simulink model "GliderSim"  (R2017a)
settings: Solver=ode4  StartTime=0.0  StopTime=10.0  FixedStep=0.01  RelTol=1e-3
libraries: simulink x1
settings Model: Creator=Caleb  LastModifiedBy=Caleb
settings DebuggingCC: AlgebraicLoopMsg=none

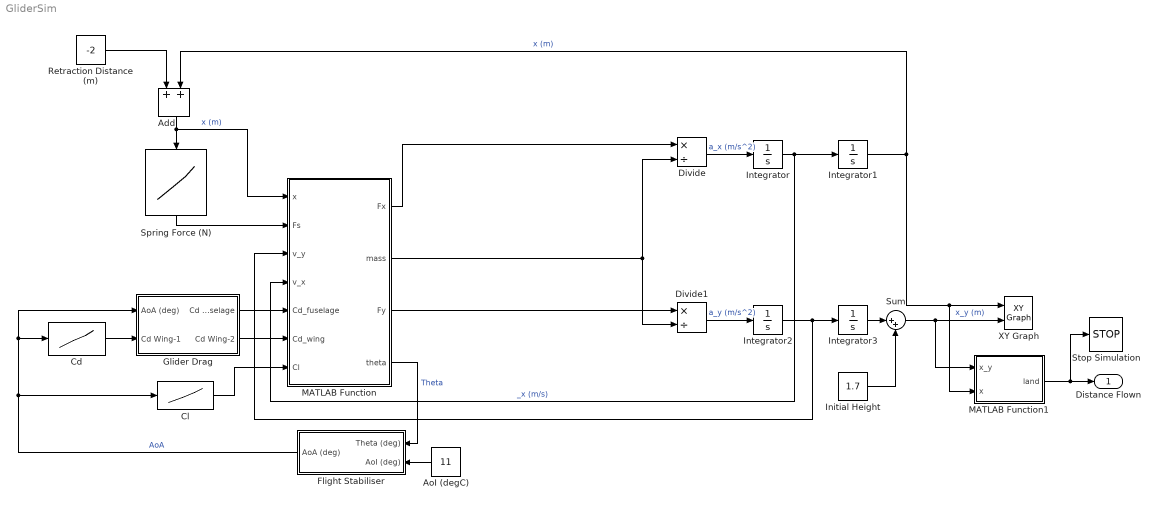
== system GliderSim ==
  Add : Sum
  AoI (degC) : Constant  Value=11
  Cd : Lookup_n-D  NumberOfTableDimensions=1  BreakpointsForDimension1="[-7.25           -7        -6.75         -6.5        -6.25           -6        -5.75         -5.5           -5        -4.75         -4.5        -4.25           -4        -3.75         -3.5        -3.25           -3        -2.75         -2.5        -2.25           -2        -1.75         -1.5        -1.25           -1        -0.75         -0.5        -0.25            0         0.25          0.5         0.75            1         1.25          1.5         1.75            2         2.25          2.5         2.75            3         3.25          3.5         3.75            4         4.25          4.5         4.75            5         5.25          5.5         5.75            6         6.25          6.5         6.75            7         7.25          7.5         7.75            8         8.25          8.5         8.75            9         9.25          9.5         9.75           10        10.25         10.5        10.75           11        11.25         11.5        11.75           12]"  Table="[0.09777      0.0974     0.09689     0.09609     0.09351     0.08904     0.08679     0.08458     0.07885     0.07578      0.0702      0.0665     0.06176     0.05768     0.05386     0.04963     0.04581     0.03137     0.02739     0.02531     0.02361     0.02247     0.02137     0.02112     0.02128     0.02105     0.02044      0.0201     0.01838     0.01859     0.01848     0.01875     0.01858     0.01891     0.01914     0.01911     0.01941     0.01899     0.01894     0.01863     0.01831     0.01814     0.01808     0.01797     0.01811     0.01819     0.01799     0.01697     0.01665     0.01637     0.01647     0.01697     0.01902     0.02138     0.02345     0.02462     0.02592     0.02747     0.02917     0.03059     0.03229      0.0344     0.03757     0.04309     0.04367     0.04789      0.0548     0.05508     0.05989     0.06817      0.0736     0.06647     0.07095      0.0758      0.0812     0.08707     0.09323]"  InternalRulePriority=Speed  RndMeth=Simplest  InputSameDT=on
  Cl : Lookup_n-D  NumberOfTableDimensions=1  BreakpointsForDimension1="[-7.25           -7        -6.75         -6.5        -6.25           -6        -5.75         -5.5           -5        -4.75         -4.5        -4.25           -4        -3.75         -3.5        -3.25           -3        -2.75         -2.5        -2.25           -2        -1.75         -1.5        -1.25           -1        -0.75         -0.5        -0.25            0         0.25          0.5         0.75            1         1.25          1.5         1.75            2         2.25          2.5         2.75            3         3.25          3.5         3.75            4         4.25          4.5         4.75            5         5.25          5.5         5.75            6         6.25          6.5         6.75            7         7.25          7.5         7.75            8         8.25          8.5         8.75            9         9.25          9.5         9.75           10        10.25         10.5        10.75           11        11.25         11.5        11.75           12]"  Table="[-0.3365     -0.3541     -0.3685     -0.3775     -0.3798     -0.3786     -0.3789     -0.3791     -0.3645     -0.3584     -0.3039     -0.2799      -0.238     -0.1968     -0.1591     -0.1118     -0.0705      0.0097      0.0582      0.0957      0.1363      0.1724       0.213       0.247      0.2882      0.3178      0.3638       0.393      0.4499      0.4792      0.5222      0.5478      0.5899      0.6131      0.6407      0.6755         0.7      0.7402      0.7667      0.7963      0.8258       0.854      0.8828      0.9128      0.9373      0.9628      0.9903      1.0184      1.0395      1.0579      1.0721      1.0813      1.0773      1.0773      1.0819      1.0965      1.1091      1.1174      1.1213      1.1304      1.1416      1.1651      1.2133      1.2732      1.2909       1.315       1.345        1.34      1.3474       1.347       1.319      1.2176      1.1873      1.1566      1.1247      1.0927      1.0614]"  InternalRulePriority=Speed  RndMeth=Simplest  InputSameDT=on
  Divide : Product  Inputs=*/
  Divide1 : Product  Inputs=*/
  Flight Stabiliser : Subsystem
  Glider Drag : Subsystem
  Initial Height : Constant  Value=1.7
  Integrator{,1..3} (4 alike) : Integrator
  MATLAB Function : MATLAB Function  TreatAsAtomicUnit=on
  MATLAB Function1 : MATLAB Function  TreatAsAtomicUnit=on
  Retraction Distance (m) : Constant  Value=-2
  Spring Force (N) : Lookup_n-D  NumberOfTableDimensions=1  BreakpointsForDimension1=[-2.16;-1.86;-1.62;-1.32;-1.00;-0.78;-0.42;-0.20;0;1]  Table=[75;62;56;48;40;33;23;13;0;0]  InternalRulePriority=Speed  RndMeth=Simplest  InputSameDT=on
  Stop Simulation : Stop
  Sum : Sum  Inputs=|++
  XY Graph : simulink/Sinks/XY Graph  xmin=0  xmax=70  ymin=0  ymax=5  st=-1
  Distance Flown : Outport
  wires:
  Add/1 -> MATLAB Function/1(x), Spring Force (N)/1  "x (m)"
  Divide/1 -> Integrator/1  "a_x (m/s^2)"
  Integrator/1 -> Integrator1/1, MATLAB Function/4(v_x)  "_x (m/s)"
  Integrator1/1 -> MATLAB Function1/2(x), XY Graph/1, Add/2  "x (m)"
  Retraction Distance (m)/1 -> Add/1
  Spring Force (N)/1 -> MATLAB Function/2(Fs)
  MATLAB Function/1(Fx) -> Divide/1
  MATLAB Function/2(mass) -> Divide/2, Divide1/2
  MATLAB Function/3(Fy) -> Divide1/1
  Divide1/1 -> Integrator2/1  "a_y (m/s^2)"
  Integrator2/1 -> Integrator3/1, MATLAB Function/3(v_y)
  Integrator3/1 -> Sum/1
  Initial Height/1 -> Sum/2
  Sum/1 -> XY Graph/2, MATLAB Function1/1(x_y)  "x_y (m)"
  MATLAB Function1/1(land) -> Stop Simulation/1, Distance Flown/1
  Flight Stabiliser/1(AoA (deg)) -> Glider Drag/1(AoA (deg)), Cd/1, Cl/1  "AoA"
  MATLAB Function/4(theta) -> Flight Stabiliser/1(Theta (deg))  "Theta"
  Cl/1 -> MATLAB Function/7(Cl)
  AoI (degC)/1 -> Flight Stabiliser/2(AoI (deg))
  Cd/1 -> Glider Drag/2(Cd Wing-1)
  Glider Drag/2(Cd Wing-2) -> MATLAB Function/6(Cd_wing)
  Glider Drag/1(Cd Fuselage) -> MATLAB Function/5(Cd_fuselage)

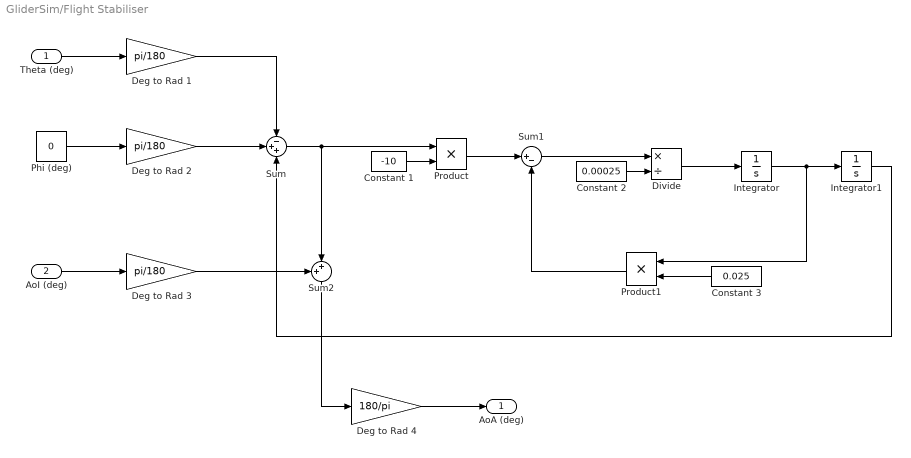
== system GliderSim/Flight Stabiliser ==
  Theta (deg) : Inport
  AoI (deg) : Inport  Port=2
  Constant 1 : Constant  Value=-10
  Constant 2 : Constant  Value=0.00025
  Constant 3 : Constant  Value=0.025
  Deg to Rad 1 : Gain  Gain=pi/180
  Deg to Rad 2 : Gain  Gain=pi/180
  Deg to Rad 3 : Gain  Gain=pi/180
  Deg to Rad 4 : Gain  Gain=180/pi
  Divide : Product  Inputs=*/
  Integrator : Integrator
  Integrator1 : Integrator
  Phi (deg) : Constant  Value=0
  Product : Product
  Product1 : Product
  Sum : Sum  Inputs=-++
  Sum1 : Sum  Inputs=|+-
  Sum2 : Sum  Inputs=++|
  AoA (deg) : Outport
  wires:
  Sum/1 -> Sum2/2, Product/1
  Divide/1 -> Integrator/1
  Integrator/1 -> Product1/1, Integrator1/1
  Sum1/1 -> Divide/1
  Deg to Rad 2/1 -> Sum/2
  Constant 1/1 -> Product/2
  Product/1 -> Sum1/1
  Constant 2/1 -> Divide/2
  Phi (deg)/1 -> Deg to Rad 2/1
  Sum2/1 -> Deg to Rad 4/1
  Deg to Rad 3/1 -> Sum2/1
  Theta (deg)/1 -> Deg to Rad 1/1
  AoI (deg)/1 -> Deg to Rad 3/1
  Product1/1 -> Sum1/2
  Integrator1/1 -> Sum/3
  Constant 3/1 -> Product1/2
  Deg to Rad 1/1 -> Sum/1
  Deg to Rad 4/1 -> AoA (deg)/1

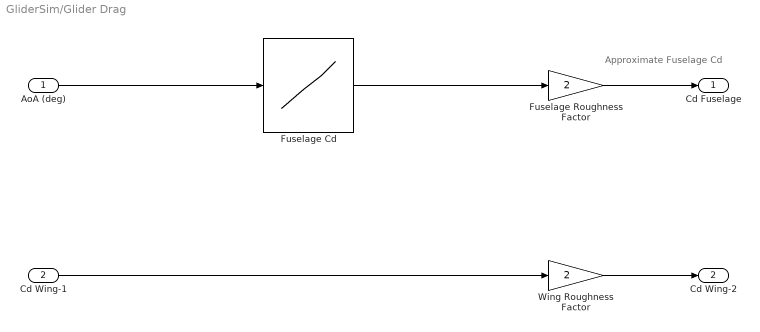
== system GliderSim/Glider Drag ==
  note: Approximate
      | Fuselage Cd
  AoA (deg) : Inport
  Cd Wing-1 : Inport  Port=2
  Fuselage Roughness Factor : Gain  Gain=2
  Fuselage Cd : Lookup_n-D  NumberOfTableDimensions=1  BreakpointsForDimension1=|  Table=|  InternalRulePriority=Speed  RndMeth=Simplest  InputSameDT=on
      BreakpointsForDimension1=|
      | [-20
      | -18
      | -16
      | -14
      | -12
      | -10
      | -8
      | -6
      | -5
      | -4
      | -2
      | 0
      | 2
      | 4
      | 6
      | 8
      | 10
      | 12
      | 14
      | 16
      | 18
      | 20]
      Table=|
      | [6.450028
      | 5.279805
      | 4.3229889
      | 3.2581778
      | 3.11992
      | 2.0828604
      | 1.4706347
      | 1.1015511
      | 0.94659083
      | 0.85580422
      | 0.73686307
      | 0.61427749
      | 0.75004173
      | 0.86217343
      | 1.1007998
      | 1.471149
      | 2.0086569
      | 3.0671467
      | 3.2583681
      | 4.2917072
      | 5.3059248
      | 6.3925707]
  Wing Roughness Factor : Gain  Gain=2
  Cd Fuselage : Outport
  Cd Wing-2 : Outport  Port=2
  wires:
  Wing Roughness Factor/1 -> Cd Wing-2/1
  Cd Wing-1/1 -> Wing Roughness Factor/1
  Fuselage Roughness Factor/1 -> Cd Fuselage/1
  AoA (deg)/1 -> Fuselage Cd/1
  Fuselage Cd/1 -> Fuselage Roughness Factor/1

== matlab function GliderSim/MATLAB Function1 ==
  data: x_y input; land output; x input
function land = fcn(x_y, x)

if x_y > 0
    land = 0;
else
    land = x;
end

== matlab function GliderSim/MATLAB Function ==
  data: x input; Fx output; Fs input; v_y input; v_x input; mass output; Fy output; theta output; Cd_fuselage input; Cd_wing input; Cl input
function [Fx, mass, Fy, theta] = fcn(x, Fs, v_y, v_x, Cd_fuselage, Cd_wing, Cl)

Awing = 0.06;                   %wing lift/drag area (m^2)
Afuselage = 0.002875;    %fuselage drag area(m^2)
rho = 1.225;                    %air density (kg/m^3)

msled = 0.1;            %mass of the sled (kg)
mglider = 0.021 + 0.043;%mass of glider (carbon fiber rod plus styrofoam) (kg)
mqrp = 0.03;            %mass of the QRP (kg)
mfdr = 0.018;           %mass of the FDR (kg)

g = 9.81;               %gravitional constant (m/s^2)

%drag relationship
Fd = Cd_wing*0.5*rho*Awing*v_x.^2 + Cd_fuselage*0.5*rho*Afuselage*v_x.^2;
%lift relationship
Fl = Cl*0.5*rho*Awing*v_x.^2;

V = sqrt(v_x.^2 + v_y.^2);      %resulting velocity

if x<=0
    %glider during launch
    theta = 0;                                  %angle of velocity
    mass = msled + mglider + mqrp + mfdr;       %mass of projectile
    Fx = Fs;                                    %force on x-axis
    Fy = 0;                                     %force on y-axis
else
    %glider during flight
    theta = atand(v_y/v_x);                     %angle of velocity
    mass = mglider + mfdr;                      %mass of projectile
    Fg = mass*g;                                %force from gravity
    Fx = -Fl*sind(theta)-Fd*cosd(theta);                       %force in x-axis
    Fy = Fl*cosd(theta)-Fd*sind(theta) - Fg;                  %force on y-axis
end
